simulink model "myROScomm"  (R2018b)
settings: Solver=FixedStepAuto  StartTime=0.0  StopTime=Inf  RelTol=1e-3  EnableMultiTasking=on
undefined symbols (not defined in the file): FifthOutput, MotorOutput, SteerOutput
libraries: robotlib x3
settings Model: Creator=nate  LastModifiedBy=nate
settings SolverCC: PositivePriorityOrder=on
settings OptimizationCC: EnhancedBackFolding=on  PassReuseOutputArgsAs=Individual arguments  MaxStackSize=64  OptimizeBlockOrder=speed  DifferentSizesBufferReuse=on  OptimizationCustomize=off
settings DebuggingCC: ParameterTunabilityLossMsg=error
settings HardwareCC: ProdBitPerPointer=32  ProdBitPerSizeT=32  ProdBitPerPtrDiffT=32  ProdLargestAtomicInteger=Long  ProdLargestAtomicFloat=Double  ProdWordSize=32  ProdHWDeviceType=ARM Compatible->ARM Cortex
settings SFSimCC: MATLABDynamicMemAlloc=off
settings RTWCC: SystemTargetFile=ert.tlc  HardwareBoard=Raspberry Pi - Robot Operating System (ROS)  TLCOptions="-aInlineSetEventsForThisBaseRateFcn=TLC_FALSE -aSuppressMultiTaskScheduler=TLC_FALSE  -aRateBasedStepFcn=0"  TemplateMakefile=ert_default_tmf  GenerateReport=on  Toolchain=Catkin  BuildConfiguration=Faster Runs  IncludeHyperlinkInReport=on  LaunchReport=on  TargetLang=C++  GenerateTraceInfo=on  GenerateTraceReport=on  GenerateTraceReportSl=on  GenerateTraceReportSf=on  GenerateTraceReportEml=on
settings CodeAppCC: ForceParamTrailComments=on  IgnoreCustomStorageClasses=off  OperatorAnnotations=on  SimulinkDataObjDesc=on  SFDataObjDesc=on  InsertBlockDesc=on
settings ERTTargetCC: SupportVariableSizeSignals=on

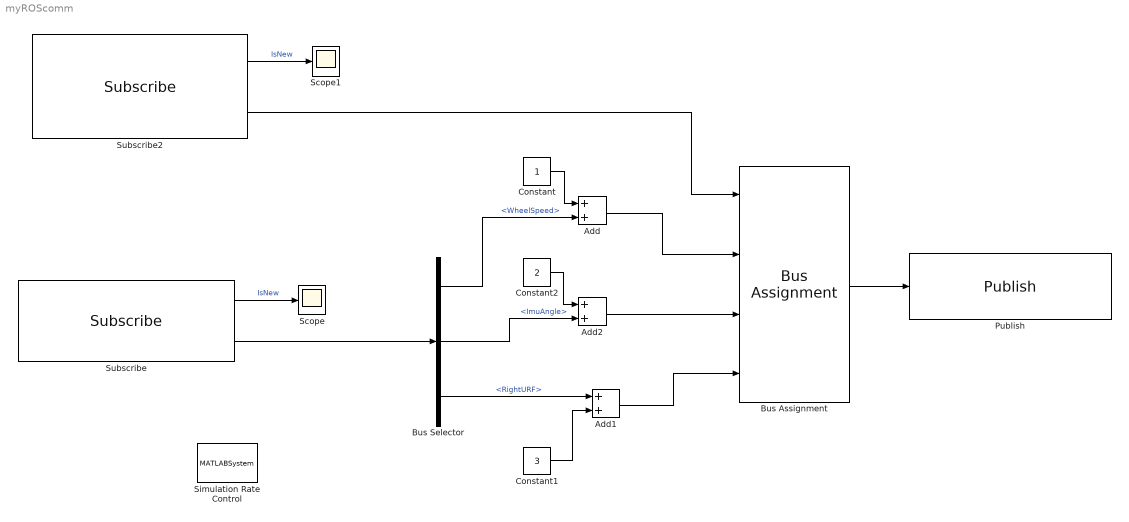
== system myROScomm ==
  Add : Sum
  Add1 : Sum
  Add2 : Sum  OutDataTypeStr=int16
  Bus Assignment : BusAssignment  AssignedSignals=MotorOutput,SteerOutput,FifthOutput
  Bus Selector : BusSelector  OutputSignals=WheelSpeed,ImuAngle,RightURF
  Constant : Constant  OutDataTypeStr=int16
  Constant1 : Constant  Value=3  OutDataTypeStr=int16
  Constant2 : Constant  Value=2  OutDataTypeStr=single
  Publish : robotlib/Publish  topicSource=Select from ROS network  topic=/pi_comm_node/teensy_actuator_data  messageType=semi_truck/Teensy_Actuators  messageQueueLength=1
      link override SinkBlock: ROSTopic=/pi_comm_node/teensy_actuator_data  ROSMessageType=semi_truck/Teensy_Actuators  SLBusName=SL_Bus_myROScomm_semi_truck_Teensy_Actuators  ModelName=myROScomm  BlockId=Pub_myROScomm_9
      settings: SourceProductBaseCode=RO
  Scope : Scope
  Scope1 : Scope
  Simulation Rate Control : MATLABSystem  System=ExampleHelperSimulationRateControl  SampleTime=0.02
      mask Type: ExampleHelperSimulationRateControl
      mask Display: disp('Rate Control');
  Subscribe : robotlib/Subscribe  topicSource=Select from ROS network  topic=/pi_comm_node/teensy_sensor_data  messageType=semi_truck/Teensy_Sensors  sampleTime=-1  messageQueueLength=51
      settings: SourceProductBaseCode=RO
  Subscribe2 : robotlib/Subscribe  topicSource=Specify your own  topic=/pi_comm_node/teensy_actuator_data  messageType=semi_truck/Teensy_Actuators  sampleTime=-1  messageQueueLength=51
      settings: SourceProductBaseCode=RO
  wires:
  Subscribe/2 -> Bus Selector/1
  Add/1 -> Bus Assignment/2
  Constant/1 -> Add/1
  Constant1/1 -> Add1/2
  Bus Assignment/1 -> Publish/1
  Constant2/1 -> Add2/1
  Bus Selector/2 -> Add2/2  "<ImuAngle>"
  Add2/1 -> Bus Assignment/3
  Add1/1 -> Bus Assignment/4
  Bus Selector/3 -> Add1/1  "<RightURF>"
  Bus Selector/1 -> Add/2  "<WheelSpeed>"
  Subscribe/1 -> Scope/1  "IsNew"
  Subscribe2/2 -> Bus Assignment/1
  Subscribe2/1 -> Scope1/1  "IsNew"
